simulink subsystem "MTPA_Field_Weakening"  (R2024a)
settings: Solver=VariableStepAuto  StartTime=0.0  StopTime=10.0  RelTol=1e-3
values from neighbouring files (symbols this model uses):
  Ismax = 2*Irated    [parameters.m]
  Lambda_m = .1821    (= 0.1821)    [parameters.m]
  Lds = .001453    (= 0.001453)    [parameters.m]
  Lqs = .001607    (= 0.001607)    [parameters.m]
  Maximum_stator_flux_linkage = Ismax*Lds    [parameters.m]
  Nm_max = Wr_max*(2/P)*(30/pi)    [parameters.m]
  P = 8    [parameters.m]
  Vsmax = Vdc/sqrt(3)    [parameters.m]
settings Model: Creator=User  LastModifiedBy=User

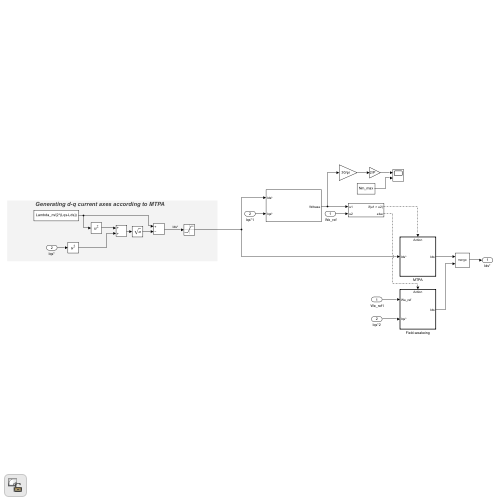
[thumbnail: Simulink's stored preview of the top-level diagram]
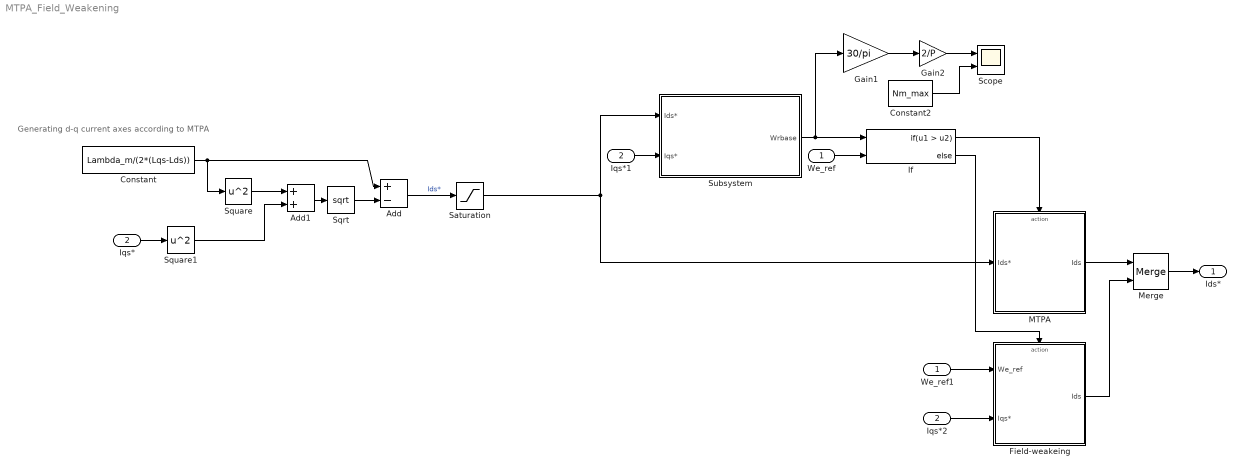
== system MTPA_Field_Weakening ==
  note: Generating d-q current axes according to MTPA
  " We_ref" : Inport
  Iqs* : Inport  Port=2
  " We_ref1" : InportShadow
  Add : Sum  Inputs=+-
  Add1 : Sum
  Constant : Constant  Value=Lambda_m/(2*(Lqs-Lds))
  Constant2 : Constant  Value=Nm_max
  Field-weakeing : Subsystem  TreatAsAtomicUnit=on
  Gain1 : Gain  Gain=30/pi
  Gain2 : Gain  Gain=2/P
  If : If  NumInputs=2  IfExpression=u1 > u2
  Iqs*1 : InportShadow  Port=2
  Iqs*2 : InportShadow  Port=2
  MTPA : Subsystem  TreatAsAtomicUnit=on
  Merge : Merge
  Saturation : Saturate  UpperLimit=0  LowerLimit=-Ismax
  Scope : Scope  NumInputPorts=2
  Sqrt : Sqrt
  Square : Math  Operator=square
  Square1 : Math  Operator=square
  Subsystem : Subsystem
  Ids* : Outport
  wires:
  Constant2/1 -> Scope/2
  Iqs*1/1 -> Subsystem/2(Iqs*)
  Gain2/1 -> Scope/1
  Constant/1 -> Square/1, Add/1
  Add1/1 -> Sqrt/1
  Square/1 -> Add1/1
  Iqs*/1 -> Square1/1
  MTPA/1(Ids) -> Merge/1
  Subsystem/1(Wrbase) -> If/1, Gain1/1
  Field-weakeing/1(Ids) -> Merge/2
  " We_ref"/1 -> If/2
  If/1 -> MTPA/Action
  " We_ref1"/1 -> Field-weakeing/1(We_ref)
  If/2 -> Field-weakeing/Action
  Sqrt/1 -> Add/2
  Square1/1 -> Add1/2
  Merge/1 -> Ids*/1
  Add/1 -> Saturation/1  "Ids*"
  Saturation/1 -> MTPA/1(Ids*), Subsystem/1(Ids*)
  Iqs*2/1 -> Field-weakeing/2(Iqs*)
  Gain1/1 -> Gain2/1

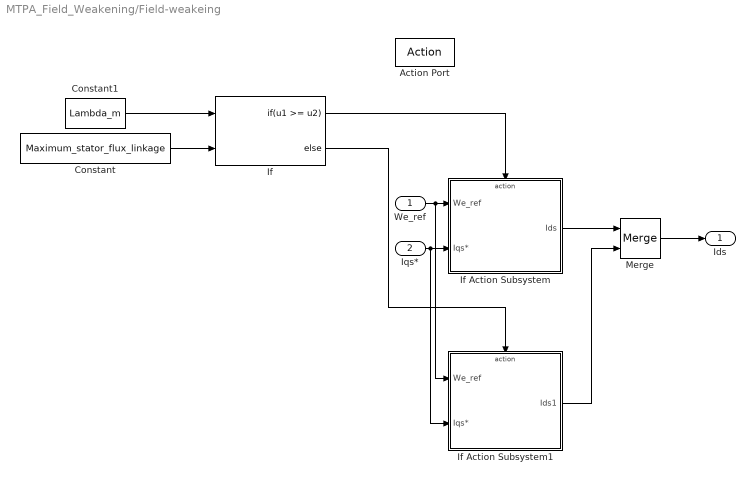
== system MTPA_Field_Weakening/Field-weakeing ==
  We_ref : Inport
  Iqs* : Inport  Port=2
  Action Port : ActionPort
  Constant : Constant  Value=Maximum_stator_flux_linkage
  Constant1 : Constant  Value=Lambda_m
  If : If  NumInputs=2  IfExpression=u1 >= u2
  If Action Subsystem : Subsystem  TreatAsAtomicUnit=on
  If Action Subsystem1 : Subsystem  TreatAsAtomicUnit=on
  Merge : Merge
  Ids : Outport
  wires:
  Merge/1 -> Ids/1
  Constant/1 -> If/2
  Constant1/1 -> If/1
  If/1 -> If Action Subsystem/Action
  We_ref/1 -> If Action Subsystem1/1(We_ref), If Action Subsystem/1(We_ref)
  Iqs*/1 -> If Action Subsystem1/2(Iqs*), If Action Subsystem/2(Iqs*)
  If/2 -> If Action Subsystem1/Action
  If Action Subsystem/1(Ids) -> Merge/1
  If Action Subsystem1/1(Ids1) -> Merge/2

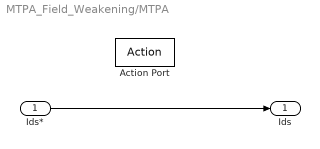
== system MTPA_Field_Weakening/MTPA ==
  Ids* : Inport
  Action Port : ActionPort
  Ids : Outport
  wires:
  Ids*/1 -> Ids/1

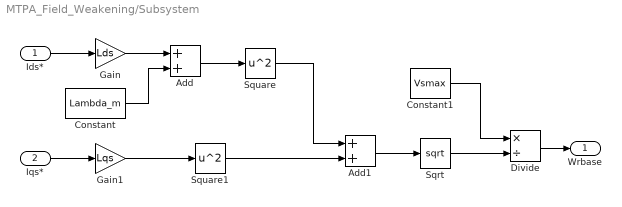
== system MTPA_Field_Weakening/Subsystem ==
  Ids* : Inport
  Iqs* : Inport  Port=2
  Add : Sum
  Add1 : Sum
  Constant : Constant  Value=Lambda_m
  Constant1 : Constant  Value=Vsmax
  Divide : Product  Inputs=*/
  Gain : Gain  Gain=Lds
  Gain1 : Gain  Gain=Lqs
  Sqrt : Sqrt
  Square : Math  Operator=square
  Square1 : Math  Operator=square
  Wrbase : Outport
  wires:
  Ids*/1 -> Gain/1
  Iqs*/1 -> Gain1/1
  Gain/1 -> Add/1
  Constant/1 -> Add/2
  Add/1 -> Square/1
  Gain1/1 -> Square1/1
  Square1/1 -> Add1/2
  Square/1 -> Add1/1
  Add1/1 -> Sqrt/1
  Sqrt/1 -> Divide/2
  Constant1/1 -> Divide/1
  Divide/1 -> Wrbase/1

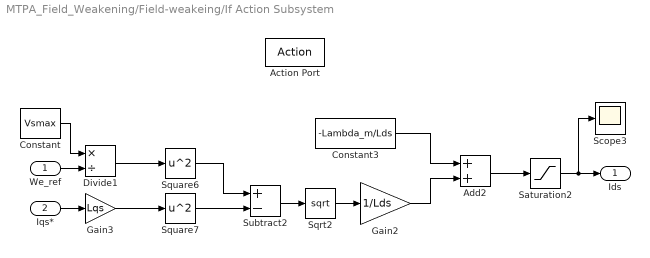
== system MTPA_Field_Weakening/Field-weakeing/If Action Subsystem ==
  We_ref : Inport
  Iqs* : Inport  Port=2
  Action Port : ActionPort
  Add2 : Sum
  Constant : Constant  Value=Vsmax
  Constant3 : Constant  Value=-Lambda_m/Lds
  Divide1 : Product  Inputs=*/
  Gain2 : Gain  Gain=1/Lds
  Gain3 : Gain  Gain=Lqs
  Saturation2 : Saturate  UpperLimit=0  LowerLimit=-Ismax  LinearizeAsGain=off
  Scope3 : Scope
  Sqrt2 : Sqrt
  Square6 : Math  Operator=square
  Square7 : Math  Operator=square
  Subtract2 : Sum  Inputs=+-
  Ids : Outport
  wires:
  Iqs*/1 -> Gain3/1
  We_ref/1 -> Divide1/2
  Constant3/1 -> Add2/1
  Gain2/1 -> Add2/2
  Sqrt2/1 -> Gain2/1
  Subtract2/1 -> Sqrt2/1
  Square6/1 -> Subtract2/1
  Divide1/1 -> Square6/1
  Constant/1 -> Divide1/1
  Square7/1 -> Subtract2/2
  Gain3/1 -> Square7/1
  Add2/1 -> Saturation2/1
  Saturation2/1 -> Ids/1, Scope3/1

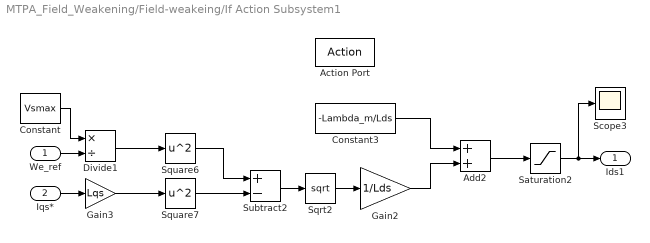
== system MTPA_Field_Weakening/Field-weakeing/If Action Subsystem1 ==
  We_ref : Inport
  Iqs* : Inport  Port=2
  Action Port : ActionPort
  Add2 : Sum
  Constant : Constant  Value=Vsmax
  Constant3 : Constant  Value=-Lambda_m/Lds
  Divide1 : Product  Inputs=*/
  Gain2 : Gain  Gain=1/Lds
  Gain3 : Gain  Gain=Lqs
  Saturation2 : Saturate  UpperLimit=0  LowerLimit=-Ismax  LinearizeAsGain=off
  Scope3 : Scope
  Sqrt2 : Sqrt
  Square6 : Math  Operator=square
  Square7 : Math  Operator=square
  Subtract2 : Sum  Inputs=+-
  Ids1 : Outport
  wires:
  Add2/1 -> Saturation2/1
  Sqrt2/1 -> Gain2/1
  Square6/1 -> Subtract2/1
  Constant/1 -> Divide1/1
  Gain3/1 -> Square7/1
  Subtract2/1 -> Sqrt2/1
  We_ref/1 -> Divide1/2
  Gain2/1 -> Add2/2
  Constant3/1 -> Add2/1
  Square7/1 -> Subtract2/2
  Iqs*/1 -> Gain3/1
  Divide1/1 -> Square6/1
  Saturation2/1 -> Ids1/1, Scope3/1
